simulink model "main_real4"  (R2023a)
settings: Solver=FixedStepAuto  StartTime=0.0  StopTime=T  FixedStep=dt  RelTol=1e-3
values from neighbouring files (symbols this model uses):
  A = -a * eye(4)    [main_real4_slx.m]    (also in main_sim2real4_slx.m; main_sim4_slx.m)
  dt = 2e-3    (= 0.002)    [main_real4_slx.m]    (also in main_sim2real4_slx.m; main_sim4_slx.m = 0.001)
  eta1 = 1e3    (= 1000)    [main_real4_slx.m]    (also in main_sim2real4_slx.m; main_sim4_slx.m)
  eta2 = 1e2    (= 100)    [main_real4_slx.m]    (also in main_sim2real4_slx.m; main_sim4_slx.m)
  n_h = 100    [main_real4_slx.m]    (also in main_sim2real4_slx.m; main_sim4_slx.m)
  n_i = 6    [main_real4_slx.m]    (also in main_sim2real4_slx.m; main_sim4_slx.m)
  n_o = 4    [main_real4_slx.m]    (also in main_sim2real4_slx.m; main_sim4_slx.m)
  rho1 = 0.0    (= 0)    [main_real4_slx.m]    (also in main_sim2real4_slx.m; main_sim4_slx.m)
  rho2 = 0.0    (= 0)    [main_real4_slx.m]    (also in main_sim2real4_slx.m; main_sim4_slx.m)
  V0 = 1e-2 * randn(n_h,n_i) + 0    [main_real4_slx.m]    (also in main_sim2real4_slx.m; main_sim4_slx.m)
  W0 = 1e-2 * randn(n_o,n_h) + 0    [main_real4_slx.m]    (also in main_sim2real4_slx.m; main_sim4_slx.m)
  X_hat_0 = X0    [main_real4_slx.m]    (also in main_sim2real4_slx.m; main_sim4_slx.m)
undefined symbols (not defined in the file or in its folder): data_003, data_004, data_005, data_2901, data_2902, I1, I1m, I2, I2m, l1, l2, lc1, lc2, m1, m2
settings Model: Creator=dding  LastModifiedBy=fairytale

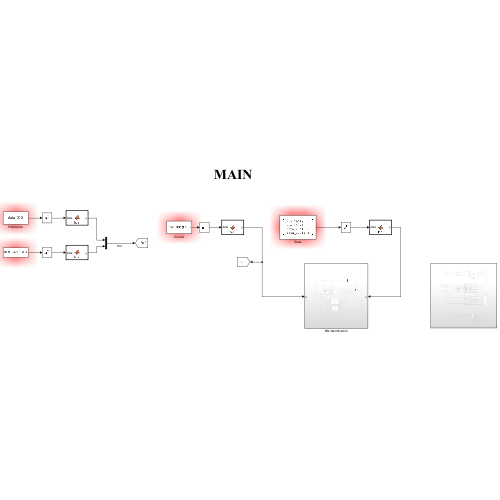
[thumbnail: Simulink's stored preview of the top-level diagram]
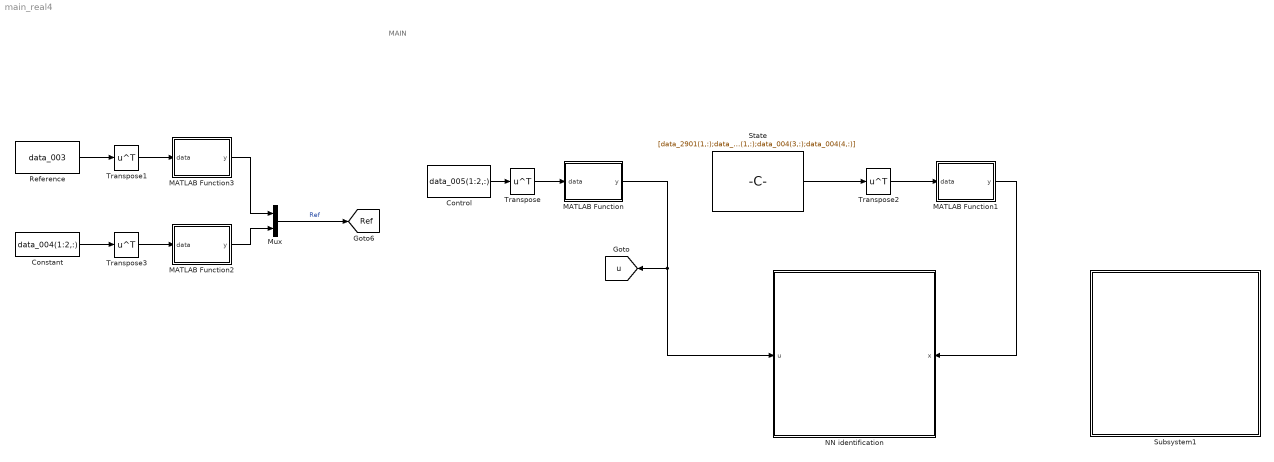
== system main_real4 ==
  note: MAIN
  Constant : Constant  Value=data_004(1:2,:)  VectorParams1D=off  SampleTime=dt
  Control : Constant  Value=data_005(1:2,:)  VectorParams1D=off  SampleTime=dt
  MATLAB Function : MATLAB Function  TreatAsAtomicUnit=on
  MATLAB Function1 : MATLAB Function  TreatAsAtomicUnit=on
  MATLAB Function2 : MATLAB Function  TreatAsAtomicUnit=on
  MATLAB Function3 : MATLAB Function  TreatAsAtomicUnit=on
  Mux : Mux  Inputs=2
  NN identification : Subsystem
      settings: PortSchema="{\"entries\":[{\"content\":{\"sides\":[{\"content\":{},\"type\":\"ConnectorPlacement.EquallySpacedRectSide\",\"uuid\":\"b5e68509-af14-483e-9022-a238da7f8976\"},{\"content\":{\"side\":\"RIGHT\"},\"type\":\"ConnectorPlacement.EquallySpacedRectSide\",\"uuid\":\"227b12d5-85c0-4871-b1f3-ce700a25cbd8\"},{\"content\":{\"connectorIds\":[\"In1\"],\"side\":\"TOP\"},\"type\":\"ConnectorPlacement.EquallySpacedRectSide\",\"uuid\":\"04532d91-bd13-4081-a0a6-2e9b5f5bbbc1\"},{\"content\":{\"connectorIds\":[\"In2\"],\"side\":\"BOTTOM\"},\"type\":\"ConnectorPlacement.EquallySpacedRectSide\",\"uuid\":\"58e23698-c698-43c7-afbb-9eb032c0630e\"}]},\"type\":\"ConnectorPlacement.EquallySpacedConnector\",\"uuid\":\"69e78e49-5ac8-44ff-82c8-e58de664d9c5\"}],\"packageUris\":[\"http://schema.mathworks.com/mf0/Connector/R2020b\"],\"version\":\"1.0\"}"
  Reference : Constant  Value=data_003  VectorParams1D=off  SampleTime=dt
  State : Constant  Value=[data_2901(1,:);data_2902(1,:);data_004(3,:);data_004(4,:)]  VectorParams1D=off  SampleTime=dt
  Subsystem1 : Subsystem
  Transpose{,1..3} (4 alike) : Math  Operator=transpose
  tag scope: Ref=global, u=global
  wires:
  Control/1 -> Transpose/1
  Transpose/1 -> MATLAB Function/1(data)
  Transpose2/1 -> MATLAB Function1/1(data)
  MATLAB Function1/1(y) -> NN identification/2(x)
  MATLAB Function/1(y) -> NN identification/1(u), [u]
  Constant/1 -> Transpose3/1
  Reference/1 -> Transpose1/1
  Transpose1/1 -> MATLAB Function3/1(data)
  Transpose3/1 -> MATLAB Function2/1(data)
  MATLAB Function3/1(y) -> Mux/1
  MATLAB Function2/1(y) -> Mux/2
  Mux/1 -> [Ref]  "Ref"
  State/1 -> Transpose2/1

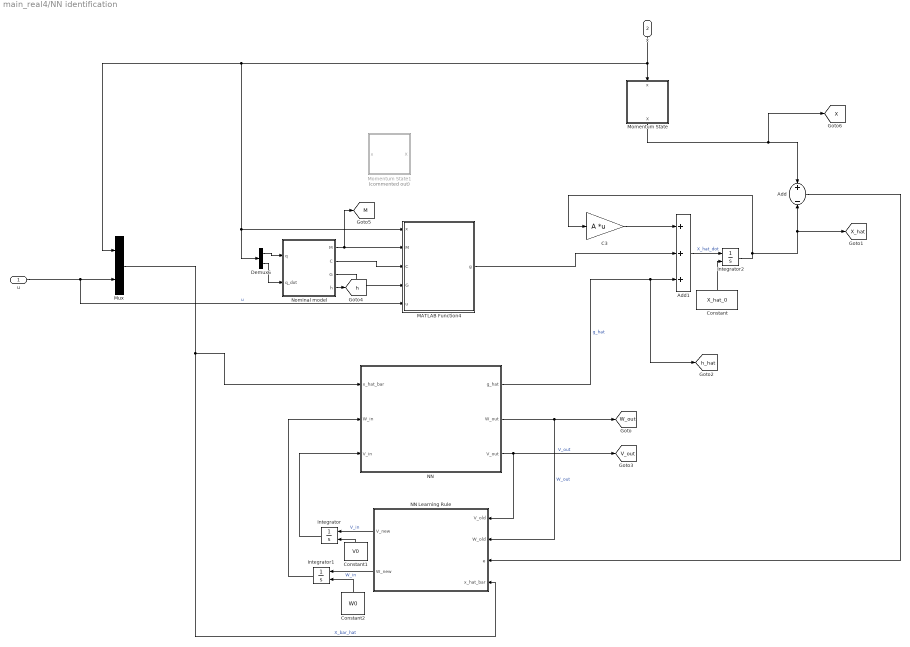
== system main_real4/NN identification ==
  u : Inport
  x : Inport  Port=2
  Add : Sum  Inputs=+-
  Add1 : Sum  Inputs=+++
  C3 : Gain  Gain=A  Multiplication=Matrix(K*u)
  Constant : Constant  Value=X_hat_0  VectorParams1D=off
  Constant1 : Constant  Value=V0  VectorParams1D=off
  Constant2 : Constant  Value=W0  VectorParams1D=off
  Demux6 : Demux  Outputs=2
  Integrator : Integrator  InitialConditionSource=external  InitialCondition=V0
  Integrator1 : Integrator  InitialConditionSource=external  InitialCondition=W0
  Integrator2 : Integrator  InitialConditionSource=external  InitialCondition=X_hat_0
  MATLAB Function4 : MATLAB Function  TreatAsAtomicUnit=on
  Momentum State : MATLAB Function  TreatAsAtomicUnit=on
  Momentum State1 : MATLAB Function  Commented=on  TreatAsAtomicUnit=on
  Mux : Mux  Inputs=2
  NN : MATLAB Function  TreatAsAtomicUnit=on
  NN Learning Rule : MATLAB Function  TreatAsAtomicUnit=on
  Nominal model : MATLAB Function  TreatAsAtomicUnit=on
  tag scope: M=global, V_out=global, W_out=global, X=global, X_hat=global, h=global, h_hat=global
  wires:
  x/1 -> Momentum State/1(x), Mux/1, MATLAB Function4/1(x), Demux6/1
  NN/2(W_out) -> [W_out], NN Learning Rule/2(W_old)  "W_out"
  Integrator2/1 -> C3/1, Add/2, [X_hat]
  Add1/1 -> Integrator2/1  "X_hat_dot"
  NN/3(V_out) -> NN Learning Rule/1(V_old), [V_out]  "V_out"
  Integrator1/1 -> NN/2(W_in)
  u/1 -> MATLAB Function4/5(u), Mux/2  "u"
  C3/1 -> Add1/1
  NN Learning Rule/1(V_new) -> Integrator/1  "V_in"
  NN Learning Rule/2(W_new) -> Integrator1/1  "W_in"
  NN/1(g_hat) -> [h_hat], Add1/3  "g_hat"
  Integrator/1 -> NN/3(V_in)
  Add/1 -> NN Learning Rule/3(e)
  Constant/1 -> Integrator2/2
  Constant2/1 -> Integrator1/2
  Constant1/1 -> Integrator/2
  Mux/1 -> NN/1(x_hat_bar), NN Learning Rule/4(x_hat_bar)  "X_bar_hat"
  Demux6/1 -> Nominal model/1(q)
  Nominal model/1(M) -> MATLAB Function4/2(M), [M]
  Nominal model/3(G) -> MATLAB Function4/4(G)
  Nominal model/2(C) -> MATLAB Function4/3(C)
  Demux6/2 -> Nominal model/2(q_dot)
  MATLAB Function4/1(g) -> Add1/2
  Momentum State/1(X) -> [X], Add/1
  Nominal model/4(h) -> [h]

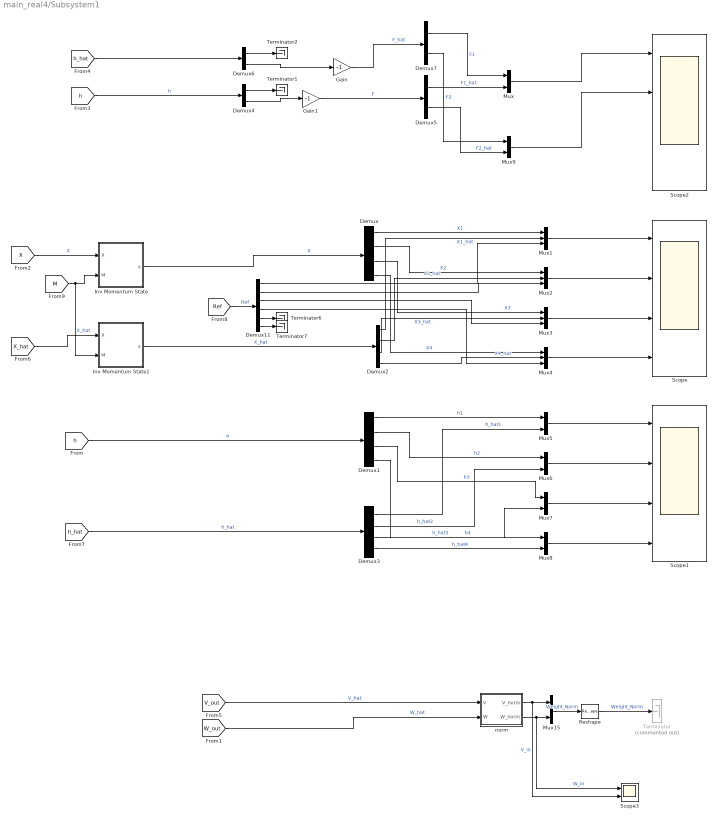
== system main_real4/Subsystem1 ==
  Demux{,1..3} (4 alike) : Demux
  Demux11 : Demux  Outputs=6
  Demux{4..7} (4 alike) : Demux  Outputs=2
  Gain : Gain  Gain=-1
  Gain1 : Gain  Gain=-1
  Inv Momentum State : MATLAB Function  TreatAsAtomicUnit=on
  Inv Momentum State1 : MATLAB Function  TreatAsAtomicUnit=on
  Mux{,5..9,15} (7 alike) : Mux  Inputs=2
  Mux{1..4} (4 alike) : Mux  Inputs=3
  Reshape : Reshape  OutputDimensionality=Column vector (2-D)
  Scope : Scope  NumInputPorts=4
  Scope1 : Scope  NumInputPorts=4
  Scope2 : Scope  NumInputPorts=4
  Scope3 : Scope  NumInputPorts=2
  Terminator : Terminator  Commented=on
  Terminator{1..2,6..7} (4 alike) : Terminator
  norm : MATLAB Function  TreatAsAtomicUnit=on
  wires:
  Demux2/2 -> Mux2/2  "X2_hat"
  Mux4/1 -> Scope/4
  Demux1/4 -> Mux8/1  "h4"
  Mux3/1 -> Scope/3
  [h_hat] -> Demux3/1  "h_hat"
  Demux3/1 -> Mux5/2  "h_hat1"
  Demux3/2 -> Mux6/2  "h_hat2"
  Demux/1 -> Mux1/1  "X1"
  [Ref] -> Demux11/1  "Ref"
  Mux5/1 -> Scope1/1
  Demux1/1 -> Mux5/1  "h1"
  Mux2/1 -> Scope/2
  Demux2/4 -> Mux4/2  "X4_hat"
  Demux/3 -> Mux3/1  "X3"
  Demux11/1 -> Mux1/3
  Mux6/1 -> Scope1/2
  Demux11/3 -> Mux3/3
  Demux11/2 -> Mux2/3
  Mux7/1 -> Scope1/3
  Demux2/1 -> Mux1/2  "X1_hat"
  Mux8/1 -> Scope1/4
  Demux2/3 -> Mux3/2  "X3_hat"
  Demux/4 -> Mux4/1  "X4"
  Demux11/6 -> Terminator7/1
  Demux/2 -> Mux2/1  "X2"
  Mux1/1 -> Scope/1
  Demux3/4 -> Mux8/2  "h_hat4"
  Demux11/5 -> Terminator6/1
  [h_hat] -> Demux6/1
  Demux1/2 -> Mux6/1  "h2"
  Demux3/3 -> Mux7/2  "h_hat3"
  Demux1/3 -> Mux7/1  "h3"
  [h] -> Demux1/1  "h"
  Demux11/4 -> Mux4/3
  Demux5/1 -> Mux/2  "F1_hat"
  Demux5/2 -> Mux9/2  "F2_hat"
  norm/1(V_norm) -> Scope3/2, Mux15/1  "V_in"
  Reshape/1 -> Terminator/1  "Weight_Norm"
  norm/2(W_norm) -> Scope3/1, Mux15/2  "W_in"
  Mux15/1 -> Reshape/1  "Weight_Norm"
  [W_out] -> norm/2(W)  "W_hat"
  [V_out] -> norm/1(V)  "V_hat"
  [h] -> Demux4/1  "h"
  Demux4/1 -> Terminator1/1
  Demux6/1 -> Terminator2/1
  Demux6/2 -> Gain/1
  Demux4/2 -> Gain1/1
  Gain1/1 -> Demux5/1  "F"
  Gain/1 -> Demux7/1  "F_hat"
  Demux7/1 -> Mux/1  "F1"
  Demux7/2 -> Mux9/1  "F2"
  Mux/1 -> Scope2/1
  Mux9/1 -> Scope2/2
  [X] -> Inv Momentum State/1(X)  "X"
  [X_hat] -> Inv Momentum State1/1(X)  "X_hat"
  Inv Momentum State/1(x) -> Demux/1  "X"
  Inv Momentum State1/1(x) -> Demux2/1  "X_hat"
  [M] -> Inv Momentum State1/2(M), Inv Momentum State/2(M)

== matlab function main_real4/NN identification/Momentum State1 ==
  data: x input; X output; m1 parameter; m2 parameter; l1 parameter; l2 parameter; lc1 parameter; lc2 parameter; I1 parameter; I2 parameter; I1m parameter; I2m parameter
function X = fcn(x, m1, m2, l1, l2, lc1, lc2, I1, I2, I1m, I2m)

    M = Inertia_M(x(1:2), x(3:4), m1, m2, l1, l2, lc1, lc2, I1, I2, I1m, I2m);
    
    X = [x(1:2); M * x(3:4)];

end



function M = Inertia_M(q, q_dot, m1, m2, l1, l2, lc1, lc2, I1, I2, I1m, I2m)
    %%
    q1 = q(1); q2 = q(2);
    q_dot1 = q_dot(1); q_dot2 = q_dot(2); 
  
    g = 9.81;    
    %%
    Mmat11=I1+I2+lc1^2*m1+l1^2*m2+lc2^2*m2+2*l1*lc2*m2*cos(q2) + I1m;
    Mmat12=I2+lc2^2*m2+l1*lc2*m2*cos(q2);
    Mmat21=I2+lc2^2*m2+l1*lc2*m2*cos(q2);
    Mmat22=I2+lc2^2*m2 + I2m;
    
    %%
    M = [
        Mmat11 Mmat12
        Mmat21 Mmat22  
        ];

end

== matlab function main_real4/NN identification/NN ==
  data: x_hat_bar input; g_hat output size=[4 1]; W_in input; W_out output; V_in input; V_out output; n_o parameter; n_i parameter; n_h parameter
function [g_hat,W_out,V_out] = NN(x_hat_bar, W_in,V_in, n_o, n_i, n_h)
    
    V_hat = V_in;
    W_hat = W_in;
    g_hat = W_hat * activate(V_hat * x_hat_bar);
    W_out = W_in;
    V_out = V_in;

end

function sigma = activate(x)
    % sigma = tanh(x) + 2*ones(size(x));
    sigma = tanh(x);
end

== matlab function main_real4/NN identification/NN Learning Rule ==
  data: V_old input; V_new output; W_new output; W_old input; e input; x_hat_bar input; A parameter; eta1 parameter; eta2 parameter; rho1 parameter; rho2 parameter; n_h parameter
function [V_new,W_new] = learningrule(V_old, W_old, e, x_hat_bar, A, eta1, eta2, rho1, rho2, n_h)

    W_hat = W_old;
    V_hat = V_old;
    
    % identification
    x_tilde = e;
    
    Lambda = zeros(n_h,n_h);
    Lambda = diag(tanh(V_hat * x_hat_bar).^2);
    
    % update the weights
    W_hat_dot = - eta1 * (x_tilde' * inv(A))' * activate(V_hat*x_hat_bar)' - rho1 * norm(x_tilde) * W_hat;
    V_hat_dot = - eta2 * (x_tilde' * inv(A) * W_hat * (eye(size(Lambda)) - Lambda))' * x_hat_bar' - rho2 * norm(x_tilde) * V_hat;
    
    W_new = W_hat_dot;
    V_new = V_hat_dot;

end

function sigma = activate(x)
    % sigma = tanh(x) + 2*ones(size(x));
    sigma = tanh(x);
end

== matlab function main_real4/NN identification/Nominal model ==
  data: q input; M output; C output; q_dot input; G output; params parameter; h output
function [M, C, G, h] = Nominal_model(q, q_dot, params)
    %%
    q1 = q(1); q2 = q(2);
    q_dot1 = q_dot(1); q_dot2 = q_dot(2); 
    
    m1 = params.m1;  m2 = params.m2;
    l1 = params.l1;  l2 = params.l2;
    lc1 = params.lc1;  lc2 = params.lc2;
    I1 = params.I1;  I2 = params.I2;
    I1m = params.I1m; I2m = params.I2m;
    b1 = params.b1;  b2 = params.b2;
    fc1 = params.fc1; fc2 = params.fc2;
    k1 = params.k1;  k2 = params.k2;

    g = 9.81;    
    %%
    Mmat11=I1+I2+lc1^2*m1+l1^2*m2+lc2^2*m2+2*l1*lc2*m2*cos(q2) + I1m;
    Mmat12=I2+lc2^2*m2+l1*lc2*m2*cos(q2);
    Mmat21=I2+lc2^2*m2+l1*lc2*m2*cos(q2);
    Mmat22=I2+lc2^2*m2 + I2m;
    
    Cmat11=(-1)*l1*lc2*m2*sin(q2)*q_dot2;
    Cmat12=(-1)*l1*lc2*m2*sin(q2)*(q_dot1+q_dot2);
    Cmat21=l1.*lc2*m2*sin(q2)*q_dot1;
    Cmat22=0;
    
    Gmat1=g*((lc1*m1+l1*m2)*cos(q1)+lc2*m2*cos(q1+q2));
    Gmat2=g*lc2*m2*cos(q1+q2);
    
    
    Fmat1=b1*tanh(k1*q_dot1)+fc1*q_dot1;
    Fmat2=b2*tanh(k2*q_dot2)+fc2*q_dot2;
    
    
    %%
    M = [
        Mmat11 Mmat12
        Mmat21 Mmat22  
        ];
    C = [
        Cmat11 Cmat12
        Cmat21 Cmat22  
        ];
    G = [
        Gmat1
        Gmat2
        ];

    F = [
        Fmat1
        Fmat2
        ];   

    h = [zeros(2,1);-F];

end

== matlab function main_real4/Subsystem1/Inv Momentum State ==
  data: X input; x output; M input
function x = fcn(X, M)

    x = [X(1:2); M \ X(3:4)];

end

== matlab function main_real4/Subsystem1/Inv Momentum State1 ==
  data: X input; x output; M input
function x = fcn(X, M)

    x = [X(1:2); M \ X(3:4)];

end

== matlab function main_real4/MATLAB Function ==
  data: data input; y output
function y = fcn(data)
% data: [N×D] 입력 (예: [12499×4])
% output: y = D×1 벡터 (각 column)

persistent idx N
if isempty(idx)
    idx = 1;
    N = size(data,1);
end

if idx > N
    y = zeros(size(data,2),1);
else
    y = data(idx,:)';  % transpose to column vector
    idx = idx + 1;
end

== matlab function main_real4/Subsystem1/norm ==
  data: V input; V_norm output; W_norm output; W input
function [V_norm,W_norm] = Norm(V, W)

    V_norm = norm(V,'fro');
    W_norm = norm(W, 'fro');
end

== matlab function main_real4/MATLAB Function1 ==
  data: data input; y output
function y = fcn(data)
% data: [N×D] 입력 (예: [12499×4])
% output: y = D×1 벡터 (각 column)

persistent idx N
if isempty(idx)
    idx = 1;
    N = size(data,1);
end

if idx > N
    y = zeros(size(data,2),1);
else
    y = data(idx,:)';  % transpose to column vector
    idx = idx + 1;
end

== matlab function main_real4/MATLAB Function2 ==
  data: data input; y output
function y = fcn(data)
% data: [N×D] 입력 (예: [12499×4])
% output: y = D×1 벡터 (각 column)

persistent idx N
if isempty(idx)
    idx = 1;
    N = size(data,1);
end

if idx > N
    y = zeros(size(data,2),1);
else
    y = data(idx,:)';  % transpose to column vector
    idx = idx + 1;
end

== matlab function main_real4/MATLAB Function3 ==
  data: data input; y output
function y = fcn(data)
% data: [N×D] 입력 (예: [12499×4])
% output: y = D×1 벡터 (각 column)

persistent idx N
if isempty(idx)
    idx = 1;
    N = size(data,1);
end

if idx > N
    y = zeros(size(data,2),1);
else
    y = data(idx,:)';  % transpose to column vector
    idx = idx + 1;
end

== matlab function main_real4/NN identification/MATLAB Function4 ==
  data: x input; M input; C input; G input; u input; g output; A parameter
function g = fcn(x,M,C,G,u,A)


    f = [x(3:4)
         C' * x(3:4) - G + u];

    X = [x(1:2)
         M * x(3:4)];

    g = f - A * X;

end

== matlab function main_real4/NN identification/Momentum State ==
  data: x input; X output; params parameter
function X = fcn(x, params)

    M = Inertia_M(x(1:2), x(3:4), params);

    X = [x(1:2); M * x(3:4)];

end



function M = Inertia_M(q, q_dot, params)
    m1 = params.m1;  m2 = params.m2;
    l1 = params.l1;  l2 = params.l2;
    lc1 = params.lc1;  lc2 = params.lc2;
    I1 = params.I1;  I2 = params.I2;
    I1m = params.I1m; I2m = params.I2m;
    b1 = params.b1;  b2 = params.b2;
    fc1 = params.fc1; fc2 = params.fc2;
    k1 = params.k1;  k2 = params.k2;    
    q1 = q(1); q2 = q(2);
    q_dot1 = q_dot(1); q_dot2 = q_dot(2); 
  
    g = 9.81;    
    %%
    Mmat11=I1+I2+lc1^2*m1+l1^2*m2+lc2^2*m2+2*l1*lc2*m2*cos(q2) + I1m;
    Mmat12=I2+lc2^2*m2+l1*lc2*m2*cos(q2);
    Mmat21=I2+lc2^2*m2+l1*lc2*m2*cos(q2);
    Mmat22=I2+lc2^2*m2 + I2m;
    
    %%
    M = [
        Mmat11 Mmat12
        Mmat21 Mmat22  
        ];

end
